simulink model "RobotModel"  (R2019a)
settings: Solver=VariableStepAuto  StartTime=0.0  StopTime=100  RelTol=1e-3
InitFcn:
  | robotInit
StopFcn:
  | SLAMmap
model workspace (MAT data in the model file):
  Vout = Simulink.Signal
  Vout.DataType = 'double'
  Vout.Dimensions = -1
  Vout.DimensionsMode = 'auto'
  Vout.Complexity = 'auto'
  Vout.SampleTime = -1
  Vout.SamplingMode = 'auto'
  vIn = Simulink.Signal
  vIn.DataType = 'double'
  vIn.Dimensions = 1
  vIn.DimensionsMode = 'Fixed'
  vIn.Complexity = 'auto'
  vIn.SampleTime = -1
  vIn.SamplingMode = 'auto'
values from neighbouring files (symbols this model uses):
  b = 0.5    [neuraldata.mat]    (also in robotInit.m)
  behavior = 0    [neuraldata.mat]    (also in robotInit.m)
  goal_pos = [15 10]    [neuraldata.mat]    (also in robotInit.m = [20;30])
  min_obs_dist = 0.5    [neuraldata.mat]    (also in robotInit.m)
  P = (eye(size(K,1))-K*H)*P    [extKalmanFilter.m]    (also in neuraldata.mat = [0 0 0 0 0 0 0 0 0 0 0 0 ... (25 elements, 5x5)]; robotInit.m = zeros(5,5))
  Q = diag([0 0 0 0 0])    [extKalmanFilter.m]    (also in neuraldata.mat = [0 0 0 0 0 0 0 0 0 0 0 0 ... (25 elements, 5x5)]; robotInit.m = diag([0 0 0 0.5 0.5]))
  R = 0.005/Ts    (= 0.1)    [extKalmanFilter.m]    (also in neuraldata.mat = [0.1 0 0 0 0 0.1 0 0 0 0 0.5 0 ... (16 elements, 4x4)]; robotInit.m = diag([0.1 0.1 0.5 0.5]))
  r = 0.1    [neuraldata.mat]    (also in robotInit.m)
  sense_angles = 0:(pi/20):2*pi    [SLAMmap.m]    (also in neuraldata.mat = [0 0.157079632679 0.314159265359 0.471238898038 0.6283185307; robotInit.m = 0:(pi/20):(2*pi))
  start_pos = [20 30 0]    [neuraldata.mat]    (also in robotInit.m = [5;5;0])
  Ts = 0.05    [extKalmanFilter.m]    (also in gpsMeasurementFcn.m; neuraldata.mat; robotInit.m)
  xhat = xhat + K*resid    [extKalmanFilter.m]    (also in neuraldata.mat = [20 30 0 0 0]; robotInit.m = [start_pos;0;0])
undefined symbols (not defined in the file or in its folder): robot_pose
libraries: neural x60, mobileRoboticsLib x7
(part 1 of 3)
settings Model: Creator=bnk2pc  LastModifiedBy=bnk2pc
settings DataIOCC: LoggingToFile=on  LoggingFileName=SLAMdata

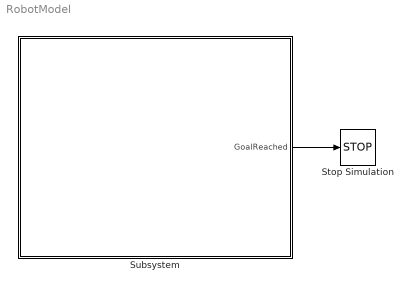
== system RobotModel ==
  Stop Simulation : Stop
  Subsystem : Subsystem
  wires:
  Subsystem/1(GoalReached) -> Stop Simulation/1

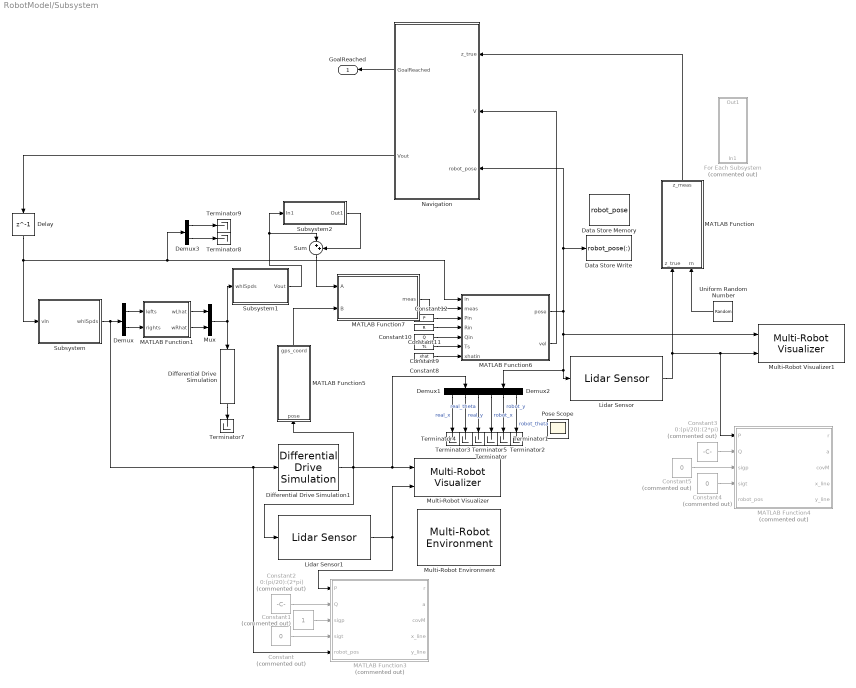
== system RobotModel/Subsystem ==
  Constant : Constant  Commented=on  Value=0
  Constant1 : Constant  Commented=on
  Constant10 : Constant  Value=Q
  Constant11 : Constant  Value=R
  Constant12 : Constant  Value=P
  Constant2 : Constant  Commented=on  Value=0:(pi/20):(2*pi)
  Constant3 : Constant  Commented=on  Value=0:(pi/20):(2*pi)
  Constant4 : Constant  Commented=on  Value=0
  Constant5 : Constant  Commented=on  Value=0
  Constant8 : Constant  Value=xhat
  Constant9 : Constant  Value=Ts
  Data Store Memory : DataStoreMemory  DataStoreName=robot_pose  ReadBeforeWriteMsg=warning  WriteAfterWriteMsg=warning  WriteAfterReadMsg=warning  InitialValue=start_pos  ShowAdditionalParam=off
  Data Store Write : DataStoreWrite  DataStoreName=robot_pose  DataStoreElements=robot_pose(:)
  Delay : Delay  DelayLength=1  InitialCondition=0
  Demux : Demux  Outputs=2
  Demux1 : Demux  Outputs=3
  Demux2 : Demux  Outputs=3
  Demux3 : Demux  Outputs=2
  Differential Drive Simulation : mobileRoboticsLib/Kinematic Models/Differential Drive/Differential Drive Simulation  wheelRadius=r  wheelBase=b  initX=start_pos(1)  initY=start_pos(2)  initAngle=start_pos(3)  Ts=Ts
      settings: SourceProductName=Mobile Robotics Simulation Toolbox
  Differential Drive Simulation1 : mobileRoboticsLib/Kinematic Models/Differential Drive/Differential Drive Simulation  wheelRadius=r  wheelBase=b  initX=start_pos(1)  initY=start_pos(2)  initAngle=start_pos(3)  Ts=Ts
      settings: SourceProductName=Mobile Robotics Simulation Toolbox
  For Each Subsystem : Subsystem  Commented=on  TreatAsAtomicUnit=on
  Lidar Sensor : mobileRoboticsLib/Environments/Lidar Sensor  mapName=map  sensorOffset=[ 0, 0 ]  scanAngles=sense_angles  maxRange=zmax
      settings: SourceProductName=Mobile Robotics Simulation Toolbox
  Lidar Sensor1 : mobileRoboticsLib/Environments/Lidar Sensor  mapName=map  sensorOffset=[ 0, 0 ]  scanAngles=sense_angles  maxRange=zmax
      settings: SourceProductName=Mobile Robotics Simulation Toolbox
  MATLAB Function : MATLAB Function  TreatAsAtomicUnit=on
  MATLAB Function1 : MATLAB Function  TreatAsAtomicUnit=on
  MATLAB Function3 : MATLAB Function  Commented=on  TreatAsAtomicUnit=on
  MATLAB Function4 : MATLAB Function  Commented=on  TreatAsAtomicUnit=on
  MATLAB Function5 : MATLAB Function  TreatAsAtomicUnit=on
  MATLAB Function6 : MATLAB Function  TreatAsAtomicUnit=on
  MATLAB Function7 : MATLAB Function  TreatAsAtomicUnit=on
  Multi-Robot Environment : mobileRoboticsLib/Environments/Multi-Robot Environment  numRobots=2  mapName=map  showWaypoints=off  showObjects=off  objectColors=[ 1, 0, 0; 0, 1, 0; 0, 0, 1 ]  objectMarkers='s'  showRobotIds=on  plotSensorLines=off
      settings: SourceProductName=Mobile Robotics Simulation Toolbox
  Multi-Robot Visualizer : mobileRoboticsLib/Environments/Multi-Robot Visualizer  idx=2  radius=0  robotColor=[1 0 0]  showTraj=on  hasLidar=on  sensorOffset=[0,0]  scanAngles=0:(pi/20):(2*pi)  maxNumScans=0  hasObjDetector=off  objDetectorOffset=[0,0]  objDetectorAngle=0  objDetectorFOV=pi/3  objDetectorMaxRange=5  hasRobotDetector=off  robotDetectorOffset=[0,0]  robotDetectorAngle=0  robotDetectorFOV=pi/3  robotDetectorMaxRange=5  robotDetectorNumDetections=0
      settings: SourceProductName=Mobile Robotics Simulation Toolbox
  Multi-Robot Visualizer1 : mobileRoboticsLib/Environments/Multi-Robot Visualizer  idx=1  radius=0  robotColor=[0 0 1]  showTraj=on  hasLidar=on  sensorOffset=[0,0]  scanAngles=0:(pi/20):(2*pi)  maxNumScans=0  hasObjDetector=off  objDetectorOffset=[0,0]  objDetectorAngle=0  objDetectorFOV=pi/3  objDetectorMaxRange=5  hasRobotDetector=off  robotDetectorOffset=[0,0]  robotDetectorAngle=0  robotDetectorFOV=pi/3  robotDetectorMaxRange=5  robotDetectorNumDetections=0
      settings: SourceProductName=Mobile Robotics Simulation Toolbox
  Mux : Mux  Inputs=2
  Navigation : Subsystem
  Pose Scope : Scope
      settings: Floating=on
  Subsystem : Subsystem
  Subsystem1 : Subsystem
  Subsystem2 : Subsystem
  Sum : Sum  Inputs=|++
  Terminator{,1..5,7..9} (9 alike) : Terminator
  Uniform Random Number : UniformRandomNumber  Minimum=0  Seed=rand  SampleTime=0.05
  GoalReached : Outport
  wires:
  Lidar Sensor/1 -> Multi-Robot Visualizer1/2, MATLAB Function4/1(P), MATLAB Function/1(z_true)
  Navigation/1(GoalReached) -> GoalReached/1
  Navigation/2("Vout ") -> Delay/1
  Delay/1 -> Subsystem/1(vIn), Demux3/1, MATLAB Function6/1(in)
  Demux/2 -> MATLAB Function1/2(rights)
  Demux/1 -> MATLAB Function1/1(lefts)
  MATLAB Function1/2(wRhat) -> Mux/2
  MATLAB Function1/1(wLhat) -> Mux/1
  Uniform Random Number/1 -> MATLAB Function/2(rn)
  Lidar Sensor1/1 -> Multi-Robot Visualizer/2, MATLAB Function3/1(P)
  Demux2/1 -> Terminator/1  "robot_x"
  Demux2/2 -> Terminator1/1  "robot_y"
  Demux2/3 -> Terminator2/1  "robot_theta"
  Demux1/1 -> Terminator3/1  "real_x"
  Demux1/2 -> Terminator4/1  "real_y"
  Demux1/3 -> Terminator5/1  "real_theta"
  Constant/1 -> MATLAB Function3/4(sigt)
  Subsystem/1(whlSpds) -> MATLAB Function3/5(robot_pos), Differential Drive Simulation1/1, Demux/1
  Constant1/1 -> MATLAB Function3/3(sigp)
  Constant2/1 -> MATLAB Function3/2(Q)
  Constant3/1 -> MATLAB Function4/2(Q)
  Constant5/1 -> MATLAB Function4/3(sigp)
  Constant4/1 -> MATLAB Function4/4(sigt)
  Differential Drive Simulation1/1 -> MATLAB Function5/1(pose), Multi-Robot Visualizer/1, Demux1/1, Lidar Sensor1/1
  Constant8/1 -> MATLAB Function6/7(xhatin)
  Constant9/1 -> MATLAB Function6/6(Ts)
  Constant10/1 -> MATLAB Function6/5(Qin)
  Constant11/1 -> MATLAB Function6/4(Rin)
  Constant12/1 -> MATLAB Function6/3(Pin)
  Mux/1 -> Differential Drive Simulation/1, Subsystem1/1(whlSpds)
  Differential Drive Simulation/1 -> Terminator7/1
  MATLAB Function5/1(gps_coord) -> MATLAB Function7/2(B)
  MATLAB Function6/1(pose) -> Multi-Robot Visualizer1/1, Demux2/1, Lidar Sensor/1, Navigation/3(robot_pose), Data Store Write/1
  MATLAB Function7/1(meas) -> MATLAB Function6/2(meas)
  MATLAB Function6/2(vel) -> Navigation/2(V)
  Subsystem1/1(Vout) -> Sum/1, Subsystem2/1(In1)
  MATLAB Function/1(z_meas) -> Navigation/1(z_true)
  Demux3/2 -> Terminator8/1
  Demux3/1 -> Terminator9/1
  Subsystem2/1(Out1) -> Sum/2
  Sum/1 -> MATLAB Function7/1(A)

== system RobotModel/Subsystem/For Each Subsystem ==
  In1 : Inport  Partition=on  PartitionDimension=1  PartitionWidth=1  PartitionOffset=0
  For Each : ForEach  DisableCoverage=on  IndexMode=One-based
  Subsystem2 : Subsystem
  Out1 : Outport  ConcatenationDimension=1
  wires:
  In1/1 -> Subsystem2/1(In)
  Subsystem2/1(Out) -> Out1/1

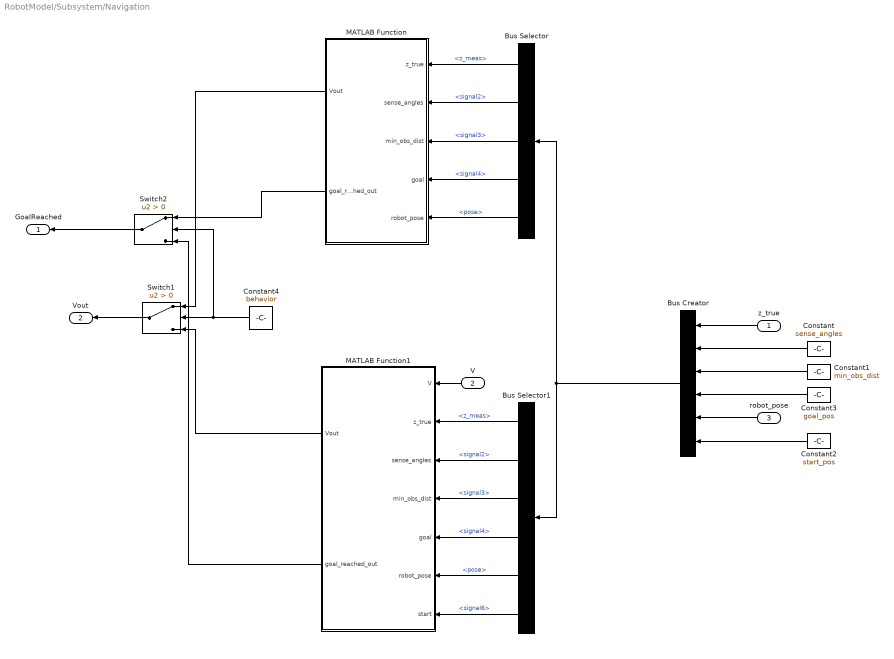
== system RobotModel/Subsystem/Navigation ==
  z_true : Inport
  V : Inport  Port=2
  robot_pose : Inport  Port=3
  Bus Creator : BusCreator  Inputs=6
  Bus Selector : BusSelector  OutputSignals=z_meas,signal2,signal3,signal4,pose
  Bus Selector1 : BusSelector  OutputSignals=z_meas,signal2,signal3,signal4,pose,signal6
  Constant : Constant  Value=sense_angles
  Constant1 : Constant  Value=min_obs_dist
  Constant2 : Constant  Value=start_pos
  Constant3 : Constant  Value=goal_pos
  Constant4 : Constant  Value=behavior
  MATLAB Function : MATLAB Function  TreatAsAtomicUnit=on
  MATLAB Function1 : MATLAB Function  TreatAsAtomicUnit=on
  Switch1 : Switch  Criteria=u2 > Threshold
  Switch2 : Switch  Criteria=u2 > Threshold
  GoalReached : Outport
  "Vout " : Outport  Port=2
  wires:
  Bus Creator/1 -> Bus Selector/1, Bus Selector1/1
  Bus Selector/1 -> MATLAB Function/1(z_true)  "<z_meas>"
  Bus Selector/2 -> MATLAB Function/2(sense_angles)  "<signal2>"
  Bus Selector/3 -> MATLAB Function/3(min_obs_dist)  "<signal3>"
  Bus Selector/4 -> MATLAB Function/4(goal)  "<signal4>"
  Bus Selector/5 -> MATLAB Function/5(robot_pose)  "<pose>"
  MATLAB Function1/1(Vout) -> Switch1/3
  Bus Selector1/1 -> MATLAB Function1/2(z_true)  "<z_meas>"
  Bus Selector1/2 -> MATLAB Function1/3(sense_angles)  "<signal2>"
  Bus Selector1/3 -> MATLAB Function1/4(min_obs_dist)  "<signal3>"
  Bus Selector1/4 -> MATLAB Function1/5(goal)  "<signal4>"
  Bus Selector1/5 -> MATLAB Function1/6(robot_pose)  "<pose>"
  V/1 -> MATLAB Function1/1(V)
  Switch1/1 -> "Vout "/1
  Constant4/1 -> Switch2/2, Switch1/2
  MATLAB Function/1(Vout) -> Switch1/1
  Switch2/1 -> GoalReached/1
  MATLAB Function/2(goal_reached_out) -> Switch2/1
  MATLAB Function1/2(goal_reached_out) -> Switch2/3
  Bus Selector1/6 -> MATLAB Function1/7(start)  "<signal6>"
  z_true/1 -> Bus Creator/1
  Constant/1 -> Bus Creator/2
  Constant1/1 -> Bus Creator/3
  Constant3/1 -> Bus Creator/4
  robot_pose/1 -> Bus Creator/5
  Constant2/1 -> Bus Creator/6

== system RobotModel/Subsystem/Subsystem ==
  vIn : Inport
  Constant6 : Constant  Value=[1/r -b/r; 1/r b/r]
  Matrix Multiply : Product  Multiplication=Matrix(*)
  whlSpds : Outport
  wires:
  Constant6/1 -> Matrix Multiply/1
  vIn/1 -> Matrix Multiply/2
  Matrix Multiply/1 -> whlSpds/1

== system RobotModel/Subsystem/Subsystem1 ==
  whlSpds : Inport
  Constant : Constant  Value=[r/2 r/2;-r/b r/b]
  Matrix Multiply : Product  Multiplication=Matrix(*)
  Vout : Outport
  wires:
  Constant/1 -> Matrix Multiply/1
  whlSpds/1 -> Matrix Multiply/2
  Matrix Multiply/1 -> Vout/1

== system RobotModel/Subsystem/Subsystem2 ==
  In1 : Inport
  Function Fitting Neural Network : Subsystem
      mask help: Function Fitting Neural Network
      mask Display: e = 0.06;c1 = [120 150 230]/255;c2 = ([120 150 230]+0)/383;c3 = ([120 150 230]+128)/383;patch([0 1 1 0],[0 0 1 1],c1);patch([0 1 1 1-e 1-e 0+e],[0 0 1 1-e 0+e 0+e],c2);patch([0 0 1 1-e 0+e 0+e],[0 1 1 1-e 1-e 0+e],c3);plot([0 1 1 0 0],[0 0 1 1 0]);fprintf('NNET');port_label('input',1,' Input');port_label('output',1,'Output ');
  Out1 : Outport
  wires:
  Function Fitting Neural Network/1(Output) -> Out1/1
  In1/1 -> Function Fitting Neural Network/1(Input)

== system RobotModel/Subsystem/For Each Subsystem/Subsystem2 ==
  In : Inport
  Pattern Recognition Neural Network : Subsystem
      mask help: Pattern Recognition Neural Network
      mask Display: e = 0.06;c1 = [120 150 230]/255;c2 = ([120 150 230]+0)/383;c3 = ([120 150 230]+128)/383;patch([0 1 1 0],[0 0 1 1],c1);patch([0 1 1 1-e 1-e 0+e],[0 0 1 1-e 0+e 0+e],c2);patch([0 0 1 1-e 0+e 0+e],[0 1 1 1-e 1-e 0+e],c3);plot([0 1 1 0 0],[0 0 1 1 0]);fprintf('NNET');port_label('input',1,' Input');port_label('output',1,'Output ');
  y1 : Scope
      mask Display: e = 0.06;c1 = [120 230 180]/255;c2 = ([120 230 180]+0)/(256+128);c3 = ([120 230 180]+128)/(256+128);patch([0 1 1 0],[0 0 1 1],c1);patch([0 1 1 1-e 1-e 0+e],[0 0 1 1-e 0+e 0+e],c2);patch([0 0 1 1-e 0+e 0+e],[0 1 1 1-e 1-e 0+e],c3);plot([0 1 1 0 0],[0 0 1 1 0]);plot([0.15 0.85 0.85 0.15 0.15],[0.5 0.5 0.85 0.85 0.5]);
  Out : Outport
  wires:
  Pattern Recognition Neural Network/1(Output) -> Out/1, y1/1
  In/1 -> Pattern Recognition Neural Network/1(Input)

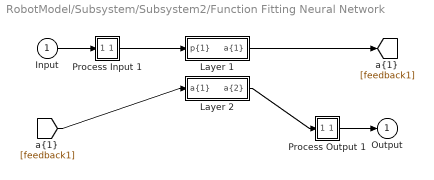
== system RobotModel/Subsystem/Subsystem2/Function Fitting Neural Network ==
  Input : Inport  PortDimensions=2
      mask Display: e = 0.06;c1 = [120 230 180]/255;c2 = ([120 230 180]+0)/(256+128);c3 = ([120 230 180]+128)/(256+128);patch([0 1 1 0],[0 0 1 1],c1);patch([0 1 1 1-e 1-e 0+e],[0 0 1 1-e 0+e 0+e],c2);patch([0 0 1 1-e 0+e 0+e],[0 1 1 1-e 1-e 0+e],c3);plot([0 1 1 0 0],[0 0 1 1 0]);
  Layer 1 : Subsystem
      mask Display: e = 0.06;c1 = [120 150 230]/255;c2 = ([120 150 230]+0)/383;c3 = ([120 150 230]+128)/383;patch([0 1 1 0],[0 0 1 1],c1);patch([0 1 1 1-e 1-e 0+e],[0 0 1 1-e 0+e 0+e],c2);patch([0 0 1 1-e 0+e 0+e],[0 1 1 1-e 1-e 0+e],c3);plot([0 1 1 0 0],[0 0 1 1 0]);
  Layer 2 : Subsystem
      mask Display: e = 0.06;c1 = [120 150 230]/255;c2 = ([120 150 230]+0)/383;c3 = ([120 150 230]+128)/383;patch([0 1 1 0],[0 0 1 1],c1);patch([0 1 1 1-e 1-e 0+e],[0 0 1 1-e 0+e 0+e],c2);patch([0 0 1 1-e 0+e 0+e],[0 1 1 1-e 1-e 0+e],c3);plot([0 1 1 0 0],[0 0 1 1 0]);
  Process Input 1 : Subsystem
      mask Display: e = 0.06;c1 = [120 150 230]/255;c2 = ([120 150 230]+0)/383;c3 = ([120 150 230]+128)/383;patch([0 1 1 0],[0 0 1 1],c1);patch([0 1 1 1-e 1-e 0+e],[0 0 1 1-e 0+e 0+e],c2);patch([0 0 1 1-e 0+e 0+e],[0 1 1 1-e 1-e 0+e],c3);plot([0 1 1 0 0],[0 0 1 1 0]);
  Process Output 1 : Subsystem
      mask Display: e = 0.06;c1 = [120 150 230]/255;c2 = ([120 150 230]+0)/383;c3 = ([120 150 230]+128)/383;patch([0 1 1 0],[0 0 1 1],c1);patch([0 1 1 1-e 1-e 0+e],[0 0 1 1-e 0+e 0+e],c2);patch([0 0 1 1-e 0+e 0+e],[0 1 1 1-e 1-e 0+e],c3);plot([0 1 1 0 0],[0 0 1 1 0]);
  Output : Outport  InitialOutput=[0;0]
      mask Display: e = 0.06;c1 = [120 230 180]/255;c2 = ([120 230 180]+0)/(256+128);c3 = ([120 230 180]+128)/(256+128);patch([0 1 1 0],[0 0 1 1],c1);patch([0 1 1 1-e 1-e 0+e],[0 0 1 1-e 0+e 0+e],c2);patch([0 0 1 1-e 0+e 0+e],[0 1 1 1-e 1-e 0+e],c3);plot([0 1 1 0 0],[0 0 1 1 0]);
  wires:
  Input/1 -> Process Input 1/1(x)
  Process Output 1/1(y) -> Output/1
  Process Input 1/1(p) -> Layer 1/1("p{1}")
  Layer 1/1("a{1}") -> [feedback1]
  [feedback1] -> Layer 2/1("a{1} ")
  Layer 2/1("a{2}") -> Process Output 1/1(a)

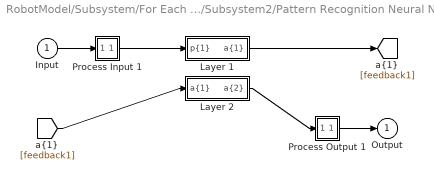
== system RobotModel/Subsystem/For Each Subsystem/Subsystem2/Pattern Recognition Neural Network ==
  Input : Inport  PortDimensions=1
      mask Display: e = 0.06;c1 = [120 230 180]/255;c2 = ([120 230 180]+0)/(256+128);c3 = ([120 230 180]+128)/(256+128);patch([0 1 1 0],[0 0 1 1],c1);patch([0 1 1 1-e 1-e 0+e],[0 0 1 1-e 0+e 0+e],c2);patch([0 0 1 1-e 0+e 0+e],[0 1 1 1-e 1-e 0+e],c3);plot([0 1 1 0 0],[0 0 1 1 0]);
  Layer 1 : Subsystem
      mask Display: e = 0.06;c1 = [120 150 230]/255;c2 = ([120 150 230]+0)/383;c3 = ([120 150 230]+128)/383;patch([0 1 1 0],[0 0 1 1],c1);patch([0 1 1 1-e 1-e 0+e],[0 0 1 1-e 0+e 0+e],c2);patch([0 0 1 1-e 0+e 0+e],[0 1 1 1-e 1-e 0+e],c3);plot([0 1 1 0 0],[0 0 1 1 0]);
  Layer 2 : Subsystem
      mask Display: e = 0.06;c1 = [120 150 230]/255;c2 = ([120 150 230]+0)/383;c3 = ([120 150 230]+128)/383;patch([0 1 1 0],[0 0 1 1],c1);patch([0 1 1 1-e 1-e 0+e],[0 0 1 1-e 0+e 0+e],c2);patch([0 0 1 1-e 0+e 0+e],[0 1 1 1-e 1-e 0+e],c3);plot([0 1 1 0 0],[0 0 1 1 0]);
  Process Input 1 : Subsystem
      mask Display: e = 0.06;c1 = [120 150 230]/255;c2 = ([120 150 230]+0)/383;c3 = ([120 150 230]+128)/383;patch([0 1 1 0],[0 0 1 1],c1);patch([0 1 1 1-e 1-e 0+e],[0 0 1 1-e 0+e 0+e],c2);patch([0 0 1 1-e 0+e 0+e],[0 1 1 1-e 1-e 0+e],c3);plot([0 1 1 0 0],[0 0 1 1 0]);
  Process Output 1 : Subsystem
      mask Display: e = 0.06;c1 = [120 150 230]/255;c2 = ([120 150 230]+0)/383;c3 = ([120 150 230]+128)/383;patch([0 1 1 0],[0 0 1 1],c1);patch([0 1 1 1-e 1-e 0+e],[0 0 1 1-e 0+e 0+e],c2);patch([0 0 1 1-e 0+e 0+e],[0 1 1 1-e 1-e 0+e],c3);plot([0 1 1 0 0],[0 0 1 1 0]);
  Output : Outport  InitialOutput=0
      mask Display: e = 0.06;c1 = [120 230 180]/255;c2 = ([120 230 180]+0)/(256+128);c3 = ([120 230 180]+128)/(256+128);patch([0 1 1 0],[0 0 1 1],c1);patch([0 1 1 1-e 1-e 0+e],[0 0 1 1-e 0+e 0+e],c2);patch([0 0 1 1-e 0+e 0+e],[0 1 1 1-e 1-e 0+e],c3);plot([0 1 1 0 0],[0 0 1 1 0]);
  wires:
  Input/1 -> Process Input 1/1(x)
  Process Output 1/1(y) -> Output/1
  Process Input 1/1(p) -> Layer 1/1("p{1}")
  Layer 1/1("a{1}") -> [feedback1]
  [feedback1] -> Layer 2/1("a{1} ")
  Layer 2/1("a{2}") -> Process Output 1/1(a)

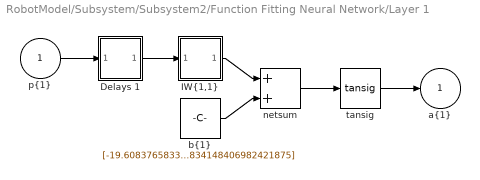
== system RobotModel/Subsystem/Subsystem2/Function Fitting Neural Network/Layer 1 ==
  "p{1}" : Inport  PortDimensions=2
      mask Display: e = 0.06;c1 = [120 230 180]/255;c2 = ([120 230 180]+0)/(256+128);c3 = ([120 230 180]+128)/(256+128);patch([0 1 1 0],[0 0 1 1],c1);patch([0 1 1 1-e 1-e 0+e],[0 0 1 1-e 0+e 0+e],c2);patch([0 0 1 1-e 0+e 0+e],[0 1 1 1-e 1-e 0+e],c3);plot([0 1 1 0 0],[0 0 1 1 0]);
  Delays 1 : Subsystem
      mask Display: e = 0.06;c1 = [120 150 230]/255;c2 = ([120 150 230]+0)/383;c3 = ([120 150 230]+128)/383;patch([0 1 1 0],[0 0 1 1],c1);patch([0 1 1 1-e 1-e 0+e],[0 0 1 1-e 0+e 0+e],c2);patch([0 0 1 1-e 0+e 0+e],[0 1 1 1-e 1-e 0+e],c3);plot([0 1 1 0 0],[0 0 1 1 0]);disp('0');
  "IW{1,1}" : Subsystem
      mask Display: e = 0.06;c1 = [120 150 230]/255;c2 = ([120 150 230]+0)/383;c3 = ([120 150 230]+128)/383;patch([0 1 1 0],[0 0 1 1],c1);patch([0 1 1 1-e 1-e 0+e],[0 0 1 1-e 0+e 0+e],c2);patch([0 0 1 1-e 0+e 0+e],[0 1 1 1-e 1-e 0+e],c3);plot([0 1 1 0 0],[0 0 1 1 0]);disp('W');
  "b{1}" : Constant  Value=[-19.608376583383943625449319370090961456298828125;23.5245751300745951084536500275135040283203125;8.26462517603339819061147863976657390594482421875;9.8552536538889814465846939128823578357696533203125;28.037670410180364655161611153744161128997802734375;-10.66542932559631395861288183368742465972900390625;-4.7206976272979250808248252724297344684600830078125;3.970651834432195048663061243132688105106353759765625;2.45723261199040710067720283404923975467681884765625;32.62803181201295643631965504027903079986572265625;-4.99971275251811508866239819326438009738922119140625;-0.447594795081393936886371420769137330353260040283203125;27.602479196059928057138677104376256465911865234375;-29.91847494412087371529196389019489288330078125;-0.3244844624488674167395174663397483527660369873046875;-9.089977152587579212195123545825481414794921875;0.4462950982925766307829462675726972520351409912109375;-0.59845995375868310528488791533163748681545257568359375;2.21575085230721935403153111110441386699676513671875;-4.92881351586324267799454901251010596752166748046875;1.9076923578129856284846255221054889261722564697265625;-40.3287955070173467220229213126003742218017578125;-1.3450935414839821913091100213932804763317108154296875;5.270636428131187045664773904718458652496337890625;0.262224879862191340151866825181059539318084716796875;9.6263684129473912065577678731642663478851318359375;4.45218514046556634866647073067724704742431640625;-10.5370708046256194023726493469439446926116943359375;1.9687509486571770356277966129709966480731964111328125;1.08443085850270204417711283895187079906463623046875;3.205132924820671913579417378059588372707366943359375;1.4027226864170436737566660667653195559978485107421875;13.2327831962293753775838922592811286449432373046875;6.1264424740605090136114085908047854900360107421875;-6.5939243507090292695238531450740993022918701171875;7.237677053105240787544971681199967861175537109375;-7.55224385878058601662132787168957293033599853515625;7.90484853977912305111885871156118810176849365234375;-8.5663464599207390648416549083776772022247314453125;-8.84304146434168814039367134682834148406982421875]
      mask Display: e = 0.06;c1 = [120 150 230]/255;c2 = ([120 150 230]+0)/383;c3 = ([120 150 230]+128)/383;patch([0 1 1 0],[0 0 1 1],c1);patch([0 1 1 1-e 1-e 0+e],[0 0 1 1-e 0+e 0+e],c2);patch([0 0 1 1-e 0+e 0+e],[0 1 1 1-e 1-e 0+e],c3);plot([0 1 1 0 0],[0 0 1 1 0]);disp('b');
  netsum : Sum  Inputs=2  SaturateOnIntegerOverflow=on  InputSameDT=on  OutDataTypeStr=Inherit: Same as first input
      mask Display: e = 0.06;c1 = [120 150 230]/255;c2 = ([120 150 230]+0)/383;c3 = ([120 150 230]+128)/383;patch([0 1 1 0],[0 0 1 1],c1);patch([0 1 1 1-e 1-e 0+e],[0 0 1 1-e 0+e 0+e],c2);patch([0 0 1 1-e 0+e 0+e],[0 1 1 1-e 1-e 0+e],c3);plot([0 1 1 0 0],[0 0 1 1 0]);disp('+');
  tansig : neural/Transfer Functions/tansig
      settings: SourceProductName=MATLAB Runtime - Deep Learning Toolbox  SourceProductBaseCode=Missing
  "a{1}" : Outport  InitialOutput=[0;0;0;0;0;0;0;0;0;0;0;0;0;0;0;0;0;0;0;0;0;0;0;0;0;0;0;0;0;0;0;0;0;0;0;0;0;0;0;0]
      mask Display: e = 0.06;c1 = [120 230 180]/255;c2 = ([120 230 180]+0)/(256+128);c3 = ([120 230 180]+128)/(256+128);patch([0 1 1 0],[0 0 1 1],c1);patch([0 1 1 1-e 1-e 0+e],[0 0 1 1-e 0+e 0+e],c2);patch([0 0 1 1-e 0+e 0+e],[0 1 1 1-e 1-e 0+e],c3);plot([0 1 1 0 0],[0 0 1 1 0]);
  wires:
  "p{1}"/1 -> Delays 1/1("p{1}")
  Delays 1/1("pd{1,1}") -> "IW{1,1}"/1("pd{1,1}")
  "IW{1,1}"/1("iz{1,1}") -> netsum/1
  "b{1}"/1 -> netsum/2
  netsum/1 -> tansig/1
  tansig/1 -> "a{1}"/1

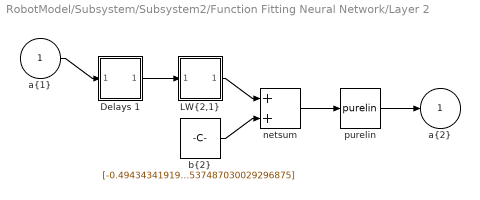
== system RobotModel/Subsystem/Subsystem2/Function Fitting Neural Network/Layer 2 ==
  "a{1} " : Inport  PortDimensions=40
      mask Display: e = 0.06;c1 = [120 230 180]/255;c2 = ([120 230 180]+0)/(256+128);c3 = ([120 230 180]+128)/(256+128);patch([0 1 1 0],[0 0 1 1],c1);patch([0 1 1 1-e 1-e 0+e],[0 0 1 1-e 0+e 0+e],c2);patch([0 0 1 1-e 0+e 0+e],[0 1 1 1-e 1-e 0+e],c3);plot([0 1 1 0 0],[0 0 1 1 0]);
  Delays 1 : Subsystem
      mask Display: e = 0.06;c1 = [120 150 230]/255;c2 = ([120 150 230]+0)/383;c3 = ([120 150 230]+128)/383;patch([0 1 1 0],[0 0 1 1],c1);patch([0 1 1 1-e 1-e 0+e],[0 0 1 1-e 0+e 0+e],c2);patch([0 0 1 1-e 0+e 0+e],[0 1 1 1-e 1-e 0+e],c3);plot([0 1 1 0 0],[0 0 1 1 0]);disp('0');
  "LW{2,1}" : Subsystem
      mask Display: e = 0.06;c1 = [120 150 230]/255;c2 = ([120 150 230]+0)/383;c3 = ([120 150 230]+128)/383;patch([0 1 1 0],[0 0 1 1],c1);patch([0 1 1 1-e 1-e 0+e],[0 0 1 1-e 0+e 0+e],c2);patch([0 0 1 1-e 0+e 0+e],[0 1 1 1-e 1-e 0+e],c3);plot([0 1 1 0 0],[0 0 1 1 0]);disp('W');
  "b{2}" : Constant  Value=[-0.494343419194449074094421803238219581544399261474609375;-0.56506799896464687815722527375328354537487030029296875]
      mask Display: e = 0.06;c1 = [120 150 230]/255;c2 = ([120 150 230]+0)/383;c3 = ([120 150 230]+128)/383;patch([0 1 1 0],[0 0 1 1],c1);patch([0 1 1 1-e 1-e 0+e],[0 0 1 1-e 0+e 0+e],c2);patch([0 0 1 1-e 0+e 0+e],[0 1 1 1-e 1-e 0+e],c3);plot([0 1 1 0 0],[0 0 1 1 0]);disp('b');
  netsum : Sum  Inputs=2  SaturateOnIntegerOverflow=on  InputSameDT=on  OutDataTypeStr=Inherit: Same as first input
      mask Display: e = 0.06;c1 = [120 150 230]/255;c2 = ([120 150 230]+0)/383;c3 = ([120 150 230]+128)/383;patch([0 1 1 0],[0 0 1 1],c1);patch([0 1 1 1-e 1-e 0+e],[0 0 1 1-e 0+e 0+e],c2);patch([0 0 1 1-e 0+e 0+e],[0 1 1 1-e 1-e 0+e],c3);plot([0 1 1 0 0],[0 0 1 1 0]);disp('+');
  purelin : neural/Transfer Functions/purelin
      settings: SourceProductName=MATLAB Runtime - Deep Learning Toolbox  SourceProductBaseCode=Missing
  "a{2}" : Outport  InitialOutput=[0;0]
      mask Display: e = 0.06;c1 = [120 230 180]/255;c2 = ([120 230 180]+0)/(256+128);c3 = ([120 230 180]+128)/(256+128);patch([0 1 1 0],[0 0 1 1],c1);patch([0 1 1 1-e 1-e 0+e],[0 0 1 1-e 0+e 0+e],c2);patch([0 0 1 1-e 0+e 0+e],[0 1 1 1-e 1-e 0+e],c3);plot([0 1 1 0 0],[0 0 1 1 0]);
  wires:
  "a{1} "/1 -> Delays 1/1("p{2}")
  Delays 1/1("pd{2,1}") -> "LW{2,1}"/1("ad{2,1}")
  "LW{2,1}"/1("lz{2,1}") -> netsum/1
  "b{2}"/1 -> netsum/2
  netsum/1 -> purelin/1
  purelin/1 -> "a{2}"/1

== system RobotModel/Subsystem/Subsystem2/Function Fitting Neural Network/Process Input 1 ==
  x : Inport  PortDimensions=2
      mask Display: e = 0.06;c1 = [120 230 180]/255;c2 = ([120 230 180]+0)/(256+128);c3 = ([120 230 180]+128)/(256+128);patch([0 1 1 0],[0 0 1 1],c1);patch([0 1 1 1-e 1-e 0+e],[0 0 1 1-e 0+e 0+e],c2);patch([0 0 1 1-e 0+e 0+e],[0 1 1 1-e 1-e 0+e],c3);plot([0 1 1 0 0],[0 0 1 1 0]);
  mapminmax : neural/Processing Functions/mapminmax  xmin=[0.189288285825714081012094425205;-45.2889527479901659035022021271]  xmax=[1.41958068528169345512424115441;45.3904770745494943184894509614]  ymin=-1  ymax=1
      settings: SourceProductName=MATLAB Runtime - Deep Learning Toolbox  SourceProductBaseCode=Missing
  p : Outport  PortDimensions=2
      mask Display: e = 0.06;c1 = [120 230 180]/255;c2 = ([120 230 180]+0)/(256+128);c3 = ([120 230 180]+128)/(256+128);patch([0 1 1 0],[0 0 1 1],c1);patch([0 1 1 1-e 1-e 0+e],[0 0 1 1-e 0+e 0+e],c2);patch([0 0 1 1-e 0+e 0+e],[0 1 1 1-e 1-e 0+e],c3);plot([0 1 1 0 0],[0 0 1 1 0]);
  wires:
  x/1 -> mapminmax/1
  mapminmax/1 -> p/1

== system RobotModel/Subsystem/Subsystem2/Function Fitting Neural Network/Process Output 1 ==
  a : Inport  PortDimensions=2
      mask Display: e = 0.06;c1 = [120 230 180]/255;c2 = ([120 230 180]+0)/(256+128);c3 = ([120 230 180]+128)/(256+128);patch([0 1 1 0],[0 0 1 1],c1);patch([0 1 1 1-e 1-e 0+e],[0 0 1 1-e 0+e 0+e],c2);patch([0 0 1 1-e 0+e 0+e],[0 1 1 1-e 1-e 0+e],c3);plot([0 1 1 0 0],[0 0 1 1 0]);
  mapminmax_reverse : neural/Processing Functions/mapminmax_reverse  xmin=[0;0]  xmax=[1;1]  ymin=-1  ymax=1
      settings: SourceProductName=MATLAB Runtime - Deep Learning Toolbox  SourceProductBaseCode=Missing
  y : Outport  PortDimensions=2
      mask Display: e = 0.06;c1 = [120 230 180]/255;c2 = ([120 230 180]+0)/(256+128);c3 = ([120 230 180]+128)/(256+128);patch([0 1 1 0],[0 0 1 1],c1);patch([0 1 1 1-e 1-e 0+e],[0 0 1 1-e 0+e 0+e],c2);patch([0 0 1 1-e 0+e 0+e],[0 1 1 1-e 1-e 0+e],c3);plot([0 1 1 0 0],[0 0 1 1 0]);
  wires:
  a/1 -> mapminmax_reverse/1
  mapminmax_reverse/1 -> y/1

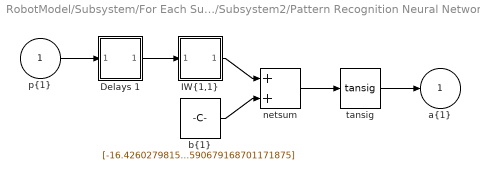
== system RobotModel/Subsystem/For Each Subsystem/Subsystem2/Pattern Recognition Neural Network/Layer 1 ==
  "p{1}" : Inport  PortDimensions=1
      mask Display: e = 0.06;c1 = [120 230 180]/255;c2 = ([120 230 180]+0)/(256+128);c3 = ([120 230 180]+128)/(256+128);patch([0 1 1 0],[0 0 1 1],c1);patch([0 1 1 1-e 1-e 0+e],[0 0 1 1-e 0+e 0+e],c2);patch([0 0 1 1-e 0+e 0+e],[0 1 1 1-e 1-e 0+e],c3);plot([0 1 1 0 0],[0 0 1 1 0]);
  Delays 1 : Subsystem
      mask Display: e = 0.06;c1 = [120 150 230]/255;c2 = ([120 150 230]+0)/383;c3 = ([120 150 230]+128)/383;patch([0 1 1 0],[0 0 1 1],c1);patch([0 1 1 1-e 1-e 0+e],[0 0 1 1-e 0+e 0+e],c2);patch([0 0 1 1-e 0+e 0+e],[0 1 1 1-e 1-e 0+e],c3);plot([0 1 1 0 0],[0 0 1 1 0]);disp('0');
  "IW{1,1}" : Subsystem
      mask Display: e = 0.06;c1 = [120 150 230]/255;c2 = ([120 150 230]+0)/383;c3 = ([120 150 230]+128)/383;patch([0 1 1 0],[0 0 1 1],c1);patch([0 1 1 1-e 1-e 0+e],[0 0 1 1-e 0+e 0+e],c2);patch([0 0 1 1-e 0+e 0+e],[0 1 1 1-e 1-e 0+e],c3);plot([0 1 1 0 0],[0 0 1 1 0]);disp('W');
  "b{1}" : Constant  Value=[-16.426027981552170587065120344050228595733642578125;-13.7350113132054172382368051330558955669403076171875;8.2006094187004858753198277554474771022796630859375;4.8358075209655932980012948974035680294036865234375;-1.5221848870557399546754595576203428208827972412109375;-1.326739256742080375062187158619053661823272705078125;-4.6401849798656957801767930504865944385528564453125;-7.77256941677534296530893698218278586864471435546875;-10.91239795844909821198598365299403667449951171875;-13.563770002615353149622023920528590679168701171875]
      mask Display: e = 0.06;c1 = [120 150 230]/255;c2 = ([120 150 230]+0)/383;c3 = ([120 150 230]+128)/383;patch([0 1 1 0],[0 0 1 1],c1);patch([0 1 1 1-e 1-e 0+e],[0 0 1 1-e 0+e 0+e],c2);patch([0 0 1 1-e 0+e 0+e],[0 1 1 1-e 1-e 0+e],c3);plot([0 1 1 0 0],[0 0 1 1 0]);disp('b');
  netsum : Sum  Inputs=2  SaturateOnIntegerOverflow=on  InputSameDT=on  OutDataTypeStr=Inherit: Same as first input
      mask Display: e = 0.06;c1 = [120 150 230]/255;c2 = ([120 150 230]+0)/383;c3 = ([120 150 230]+128)/383;patch([0 1 1 0],[0 0 1 1],c1);patch([0 1 1 1-e 1-e 0+e],[0 0 1 1-e 0+e 0+e],c2);patch([0 0 1 1-e 0+e 0+e],[0 1 1 1-e 1-e 0+e],c3);plot([0 1 1 0 0],[0 0 1 1 0]);disp('+');
  tansig : neural/Transfer Functions/tansig
      settings: SourceProductName=MATLAB Runtime - Deep Learning Toolbox  SourceProductBaseCode=Missing
  "a{1}" : Outport  InitialOutput=[0;0;0;0;0;0;0;0;0;0]
      mask Display: e = 0.06;c1 = [120 230 180]/255;c2 = ([120 230 180]+0)/(256+128);c3 = ([120 230 180]+128)/(256+128);patch([0 1 1 0],[0 0 1 1],c1);patch([0 1 1 1-e 1-e 0+e],[0 0 1 1-e 0+e 0+e],c2);patch([0 0 1 1-e 0+e 0+e],[0 1 1 1-e 1-e 0+e],c3);plot([0 1 1 0 0],[0 0 1 1 0]);
  wires:
  "p{1}"/1 -> Delays 1/1("p{1}")
  Delays 1/1("pd{1,1}") -> "IW{1,1}"/1("pd{1,1}")
  "IW{1,1}"/1("iz{1,1}") -> netsum/1
  "b{1}"/1 -> netsum/2
  netsum/1 -> tansig/1
  tansig/1 -> "a{1}"/1

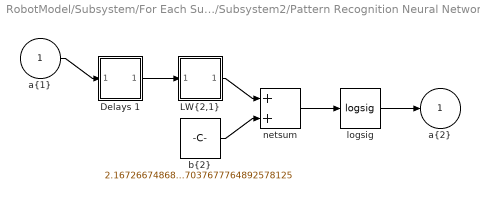
== system RobotModel/Subsystem/For Each Subsystem/Subsystem2/Pattern Recognition Neural Network/Layer 2 ==
  "a{1} " : Inport  PortDimensions=10
      mask Display: e = 0.06;c1 = [120 230 180]/255;c2 = ([120 230 180]+0)/(256+128);c3 = ([120 230 180]+128)/(256+128);patch([0 1 1 0],[0 0 1 1],c1);patch([0 1 1 1-e 1-e 0+e],[0 0 1 1-e 0+e 0+e],c2);patch([0 0 1 1-e 0+e 0+e],[0 1 1 1-e 1-e 0+e],c3);plot([0 1 1 0 0],[0 0 1 1 0]);
  Delays 1 : Subsystem
      mask Display: e = 0.06;c1 = [120 150 230]/255;c2 = ([120 150 230]+0)/383;c3 = ([120 150 230]+128)/383;patch([0 1 1 0],[0 0 1 1],c1);patch([0 1 1 1-e 1-e 0+e],[0 0 1 1-e 0+e 0+e],c2);patch([0 0 1 1-e 0+e 0+e],[0 1 1 1-e 1-e 0+e],c3);plot([0 1 1 0 0],[0 0 1 1 0]);disp('0');
  "LW{2,1}" : Subsystem
      mask Display: e = 0.06;c1 = [120 150 230]/255;c2 = ([120 150 230]+0)/383;c3 = ([120 150 230]+128)/383;patch([0 1 1 0],[0 0 1 1],c1);patch([0 1 1 1-e 1-e 0+e],[0 0 1 1-e 0+e 0+e],c2);patch([0 0 1 1-e 0+e 0+e],[0 1 1 1-e 1-e 0+e],c3);plot([0 1 1 0 0],[0 0 1 1 0]);disp('W');
  "b{2}" : Constant  Value=2.167266748688441158066098068957217037677764892578125
      mask Display: e = 0.06;c1 = [120 150 230]/255;c2 = ([120 150 230]+0)/383;c3 = ([120 150 230]+128)/383;patch([0 1 1 0],[0 0 1 1],c1);patch([0 1 1 1-e 1-e 0+e],[0 0 1 1-e 0+e 0+e],c2);patch([0 0 1 1-e 0+e 0+e],[0 1 1 1-e 1-e 0+e],c3);plot([0 1 1 0 0],[0 0 1 1 0]);disp('b');
  logsig : neural/Transfer Functions/logsig
      settings: SourceProductName=MATLAB Runtime - Deep Learning Toolbox  SourceProductBaseCode=Missing
  netsum : Sum  Inputs=2  SaturateOnIntegerOverflow=on  InputSameDT=on  OutDataTypeStr=Inherit: Same as first input
      mask Display: e = 0.06;c1 = [120 150 230]/255;c2 = ([120 150 230]+0)/383;c3 = ([120 150 230]+128)/383;patch([0 1 1 0],[0 0 1 1],c1);patch([0 1 1 1-e 1-e 0+e],[0 0 1 1-e 0+e 0+e],c2);patch([0 0 1 1-e 0+e 0+e],[0 1 1 1-e 1-e 0+e],c3);plot([0 1 1 0 0],[0 0 1 1 0]);disp('+');
  "a{2}" : Outport  InitialOutput=0
      mask Display: e = 0.06;c1 = [120 230 180]/255;c2 = ([120 230 180]+0)/(256+128);c3 = ([120 230 180]+128)/(256+128);patch([0 1 1 0],[0 0 1 1],c1);patch([0 1 1 1-e 1-e 0+e],[0 0 1 1-e 0+e 0+e],c2);patch([0 0 1 1-e 0+e 0+e],[0 1 1 1-e 1-e 0+e],c3);plot([0 1 1 0 0],[0 0 1 1 0]);
  wires:
  "a{1} "/1 -> Delays 1/1("p{2}")
  Delays 1/1("pd{2,1}") -> "LW{2,1}"/1("ad{2,1}")
  "LW{2,1}"/1("lz{2,1}") -> netsum/1
  "b{2}"/1 -> netsum/2
  netsum/1 -> logsig/1
  logsig/1 -> "a{2}"/1

== system RobotModel/Subsystem/For Each Subsystem/Subsystem2/Pattern Recognition Neural Network/Process Input 1 ==
  x : Inport  PortDimensions=1
      mask Display: e = 0.06;c1 = [120 230 180]/255;c2 = ([120 230 180]+0)/(256+128);c3 = ([120 230 180]+128)/(256+128);patch([0 1 1 0],[0 0 1 1],c1);patch([0 1 1 1-e 1-e 0+e],[0 0 1 1-e 0+e 0+e],c2);patch([0 0 1 1-e 0+e 0+e],[0 1 1 1-e 1-e 0+e],c3);plot([0 1 1 0 0],[0 0 1 1 0]);
  mapminmax : neural/Processing Functions/mapminmax  xmin=3.57448194065043478107393526422e-05  xmax=10  ymin=-1  ymax=1
      settings: SourceProductName=MATLAB Runtime - Deep Learning Toolbox  SourceProductBaseCode=Missing
  p : Outport  PortDimensions=1
      mask Display: e = 0.06;c1 = [120 230 180]/255;c2 = ([120 230 180]+0)/(256+128);c3 = ([120 230 180]+128)/(256+128);patch([0 1 1 0],[0 0 1 1],c1);patch([0 1 1 1-e 1-e 0+e],[0 0 1 1-e 0+e 0+e],c2);patch([0 0 1 1-e 0+e 0+e],[0 1 1 1-e 1-e 0+e],c3);plot([0 1 1 0 0],[0 0 1 1 0]);
  wires:
  x/1 -> mapminmax/1
  mapminmax/1 -> p/1

== system RobotModel/Subsystem/For Each Subsystem/Subsystem2/Pattern Recognition Neural Network/Process Output 1 ==
  a : Inport  PortDimensions=1
      mask Display: e = 0.06;c1 = [120 230 180]/255;c2 = ([120 230 180]+0)/(256+128);c3 = ([120 230 180]+128)/(256+128);patch([0 1 1 0],[0 0 1 1],c1);patch([0 1 1 1-e 1-e 0+e],[0 0 1 1-e 0+e 0+e],c2);patch([0 0 1 1-e 0+e 0+e],[0 1 1 1-e 1-e 0+e],c3);plot([0 1 1 0 0],[0 0 1 1 0]);
  y : Outport  PortDimensions=1
      mask Display: e = 0.06;c1 = [120 230 180]/255;c2 = ([120 230 180]+0)/(256+128);c3 = ([120 230 180]+128)/(256+128);patch([0 1 1 0],[0 0 1 1],c1);patch([0 1 1 1-e 1-e 0+e],[0 0 1 1-e 0+e 0+e],c2);patch([0 0 1 1-e 0+e 0+e],[0 1 1 1-e 1-e 0+e],c3);plot([0 1 1 0 0],[0 0 1 1 0]);
  wires:
  a/1 -> y/1

== system RobotModel/Subsystem/Subsystem2/Function Fitting Neural Network/Layer 1/Delays 1 ==
  "p{1}" : Inport  PortDimensions=2
      mask Display: e = 0.06;c1 = [120 230 180]/255;c2 = ([120 230 180]+0)/(256+128);c3 = ([120 230 180]+128)/(256+128);patch([0 1 1 0],[0 0 1 1],c1);patch([0 1 1 1-e 1-e 0+e],[0 0 1 1-e 0+e 0+e],c2);patch([0 0 1 1-e 0+e 0+e],[0 1 1 1-e 1-e 0+e],c3);plot([0 1 1 0 0],[0 0 1 1 0]);
  mux : Mux  Inputs=1
      mask Display: e = 0.06;c1 = [120 150 230]/255;c2 = ([120 150 230]+0)/383;c3 = ([120 150 230]+128)/383;patch([0 1 1 0],[0 0 1 1],c1);patch([0 1 1 1-e 1-e 0+e],[0 0 1 1-e 0+e 0+e],c2);patch([0 0 1 1-e 0+e 0+e],[0 1 1 1-e 1-e 0+e],c3);plot([0 1 1 0 0],[0 0 1 1 0]);disp('Mux')
  "pd{1,1}" : Outport
      mask Display: e = 0.06;c1 = [120 230 180]/255;c2 = ([120 230 180]+0)/(256+128);c3 = ([120 230 180]+128)/(256+128);patch([0 1 1 0],[0 0 1 1],c1);patch([0 1 1 1-e 1-e 0+e],[0 0 1 1-e 0+e 0+e],c2);patch([0 0 1 1-e 0+e 0+e],[0 1 1 1-e 1-e 0+e],c3);plot([0 1 1 0 0],[0 0 1 1 0]);
  wires:
  "p{1}"/1 -> mux/1
  mux/1 -> "pd{1,1}"/1
